simulink model "AUAV_V3_TestSensors"  (R2015a)
settings: Solver=FixedStepDiscrete  StartTime=0.0  StopTime=10.0  FixedStep=T  RelTol=1e-3
PreLoadFcn:
  | %T = 0.0025;
  | MavlinkBus;
  | mcuInit;
  | % Baro Altitude Computation
  | % =========================
  | basePressure = 98192.64;
  | baseTemp = 288.215;
  | lapseRate = -0.00198122;
  | baseHeight = 0;
undefined symbols (not defined in the file): A0, A14, A15, A2, A3, A4, A5, A6, accBiasRateLimit, apSampleTime, B0, bankCommandLimit, barAdjust, baroCutoff, baroCutTemp, baroOffset, baroScale, barTGain1, barTGain2, barTMean1, barTMean2, bda, bde, bdr, bdt, bICda, bICde, bICdr, bICdt, cubeAccelGain16405, cubeGyroGain16405, cubeMagGain16405, D0, D11, D7, D8, daLimit, data, daTrimMax, daTrimMin, deLimit, derivativesConstant, deTrimMax, deTrimMin, drLimit, drTrimMax, drTrimMin, dtLimit, dtTrimMax, dtTrimMin, F2, F3, G0, G13, G15, gaind, GS_location, gyroBiasRateLimit, IC1max, imuOffset_xacc ... (+77)
libraries: MCHP_Blockset x158, simulink x84, SLUGS_Library x31, aerolibconvert2 x6, aerolibutil x4, aerolibtransform2 x3, dspmtrx3 x2, aerolibobsolete x2
(part 17 of 23)

== system AUAV_V3_TestSensors/Sensor_Data_Adapter/Sensor Suite/Low Pass Filtering,Temperature Compensation and Calibration ==
  Baro raw : Inport
  Pitot raw : Inport  Port=2
  Power Raw : Inport  Port=3
  Therm Raw : Inport  Port=4
  Baro Altimeter : Subsystem
  Barometer Unit Conversion : Subsystem  mask{bias=baroOffset, gains=baroScale}
      mask prompts: bias "Initial Bias"; gains "Initial Gains"
      mask help: Convert Analog readings to units
  Data Type Conversion1 : DataTypeConversion  OutDataTypeStr=single
  Data Type Conversion{3,5..6,19} (4 alike) : DataTypeConversion  OutDataTypeStr=double
  Data Type Conversion4 : DataTypeConversion  OutDataTypeStr=single
  Data Type Conversion8 : DataTypeConversion  OutDataTypeStr=uint16
  Pitot Unit Conversion : Subsystem  mask{bias=pitotOffset, gains=pitotScale}
      mask prompts: bias "Initial Bias"; gains "Initial Gains"
      mask help: Convert Analog readings to units
  Power Unit Conversion : Subsystem  mask{bias=powerOffset, gains=powerScale}
      mask prompts: bias "Initial Bias"; gains "Initial Gains"
      mask help: Convert Analog readings to units
  Temp Compensate Accel X1 : Subsystem
  Temp Compensate Baro : Subsystem
  Thermistor Unit Conversion : Subsystem  mask{bias=tempOffset, gains=tempScale}
      mask prompts: bias "Initial Bias"; gains "Initial Gains"
      mask help: Convert Analog readings to units
  "Tustin Lowpass, Auto Initial Condition1" : Subsystem  mask(Tustin1stOrderLowpassAutoInitialCondition){f=lowRateSensorCutoff, T=apSampleTime}
      mask prompts: f "Lowpass Frequency"; T "Sample Time"
      mask help: Takes a 3db rolloff frequency (in Hz, NOT radians/s) and a sample time. Performs a symbolic Tustin conversion and implements in a discrete filter. The initial output of the filter is set by the first sample.
      mask Help: Enter the desired 3db rolloff frequency in Hz and the sample time. Initial conditions are sampled automatically.
      mask Display: fprintf('%.2f Hz lowpass',f)
  "Tustin Lowpass, Auto Initial Condition2" : Subsystem  mask(Tustin1stOrderLowpassAutoInitialCondition){f=lowRateSensorCutoff, T=apSampleTime}
      mask prompts: f "Lowpass Frequency"; T "Sample Time"
      mask help: Takes a 3db rolloff frequency (in Hz, NOT radians/s) and a sample time. Performs a symbolic Tustin conversion and implements in a discrete filter. The initial output of the filter is set by the first sample.
      mask Help: Enter the desired 3db rolloff frequency in Hz and the sample time. Initial conditions are sampled automatically.
      mask Display: fprintf('%.2f Hz lowpass',f)
  "Tustin Lowpass, Auto Initial Condition3" : Subsystem  mask(Tustin1stOrderLowpassAutoInitialCondition){f=pressureSensorCutoff, T=apSampleTime}
      mask prompts: f "Lowpass Frequency"; T "Sample Time"
      mask help: Takes a 3db rolloff frequency (in Hz, NOT radians/s) and a sample time. Performs a symbolic Tustin conversion and implements in a discrete filter. The initial output of the filter is set by the first sample.
      mask Help: Enter the desired 3db rolloff frequency in Hz and the sample time. Initial conditions are sampled automatically.
      mask Display: fprintf('%.2f Hz lowpass',f)
  "Tustin Lowpass, Auto Initial Condition4" : Subsystem  mask(Tustin1stOrderLowpassAutoInitialCondition){f=pressureSensorCutoff, T=apSampleTime}
      mask prompts: f "Lowpass Frequency"; T "Sample Time"
      mask help: Takes a 3db rolloff frequency (in Hz, NOT radians/s) and a sample time. Performs a symbolic Tustin conversion and implements in a discrete filter. The initial output of the filter is set by the first sample.
      mask Help: Enter the desired 3db rolloff frequency in Hz and the sample time. Initial conditions are sampled automatically.
      mask Display: fprintf('%.2f Hz lowpass',f)
  "[0.001  maxDynPress]" : Saturate  UpperLimit=maxDynPressure  LowerLimit=0.001
  Baro Alt (m) : Outport
  Pitot (Pa) : Outport  Port=2
  Static (Pa) : Outport  Port=3
  Temp (0.1 C) : Outport  Port=4
  Power (V) : Outport  Port=5
  wires:
  "Tustin Lowpass, Auto Initial Condition1"/1(Out1) -> Thermistor Unit Conversion/1(Raw)
  "[0.001  maxDynPress]"/1 -> Pitot (Pa)/1
  Data Type Conversion19/1 -> "Tustin Lowpass, Auto Initial Condition4"/1(In1)
  Data Type Conversion3/1 -> "Tustin Lowpass, Auto Initial Condition3"/1(In1)
  "Tustin Lowpass, Auto Initial Condition3"/1(Out1) -> Data Type Conversion4/1
  Data Type Conversion5/1 -> "Tustin Lowpass, Auto Initial Condition1"/1(In1)
  Therm Raw/1 -> Data Type Conversion5/1
  Barometer Unit Conversion/1(Comp) -> Static (Pa)/1, Baro Altimeter/1(Static (Pa))
  Data Type Conversion4/1 -> Pitot Unit Conversion/1(Raw)
  "Tustin Lowpass, Auto Initial Condition4"/1(Out1) -> Data Type Conversion1/1
  Data Type Conversion1/1 -> Barometer Unit Conversion/1(Raw)
  Thermistor Unit Conversion/1(Comp) -> Temp (0.1 C)/1, [Temp]
  Data Type Conversion6/1 -> "Tustin Lowpass, Auto Initial Condition2"/1(In1)
  Power Raw/1 -> Data Type Conversion6/1
  "Tustin Lowpass, Auto Initial Condition2"/1(Out1) -> Power Unit Conversion/1(Raw)
  Data Type Conversion8/1 -> Power (V)/1
  Baro Altimeter/1(Altitude) -> Baro Alt (m)/1
  Pitot Unit Conversion/1(Comp) -> "[0.001  maxDynPress]"/1
  Power Unit Conversion/1(Comp) -> Data Type Conversion8/1
  Temp Compensate Baro/1(Baro_c) -> Data Type Conversion19/1
  [Temp] -> Temp Compensate Baro/1(Temp)
  Baro raw/1 -> Temp Compensate Baro/2(Baro)
  [Temp] -> Temp Compensate Accel X1/1(Temp)
  Pitot raw/1 -> Temp Compensate Accel X1/2(Dynamic)
  Temp Compensate Accel X1/1(Baro_c) -> Data Type Conversion3/1

== system AUAV_V3_TestSensors/Trim Vals [updated 4.28.16]/Control Surface Input/2 sec  tau ==
  In1 : Inport
  Constant : Constant  Value=T
  Constant1 : Constant  Value=f
  Embedded MATLAB Function : MATLAB Function  TreatAsAtomicUnit=on
  Out1 : Outport
  wires:
  In1/1 -> Embedded MATLAB Function/1(u)
  Embedded MATLAB Function/1(y) -> Out1/1
  Constant1/1 -> Embedded MATLAB Function/3(f)
  Constant/1 -> Embedded MATLAB Function/2(T)

== system AUAV_V3_TestSensors/Trim Vals [updated 4.28.16]/Control Surface Input/2 sec  tau1 ==
  In1 : Inport
  Constant : Constant  Value=T
  Constant1 : Constant  Value=f
  Embedded MATLAB Function : MATLAB Function  TreatAsAtomicUnit=on
  Out1 : Outport
  wires:
  Constant/1 -> Embedded MATLAB Function/2(T)
  Constant1/1 -> Embedded MATLAB Function/3(f)
  Embedded MATLAB Function/1(y) -> Out1/1
  In1/1 -> Embedded MATLAB Function/1(u)

== system AUAV_V3_TestSensors/Trim Vals [updated 4.28.16]/Detect Transition High to Low/Subsystem ==
  WP Fly : Inport
  C Function Call : MCHP_Blockset/User Functions/C Function Call  ParseFilesChkbx=off  ListFunctions1=Custom Function  Function1=extern uint8_T justEnabled(uint8_T u1, uint8_T u2);  AddHeaderDeclaration=on  Function1Type=when block is updated (default)  Fct1BlockIn=u1, u2  FctReturnBlockOut=on  DataCollected=0  ORDERING=None  SampleTime=-1  MCHP_MASTERLINK=|  PinDigitalInput=[]  PinDigitalOutput=[]  PinAnalogInput=[]
      | AUAV_V3_TestSensors/Microchip Master
      | AUAV V3 Board
      | Busy Flag on D2 (RA6)
  Data Type Conversion1 : DataTypeConversion  OutDataTypeStr=uint8  SampleTime=apSampleTime
  Index : Constant  Value=2  OutDataTypeStr=uint8
  Just Enab : Outport
  wires:
  WP Fly/1 -> Data Type Conversion1/1
  Data Type Conversion1/1 -> C Function Call/1
  Index/1 -> C Function Call/2
  C Function Call/1 -> Just Enab/1

== system AUAV_V3_TestSensors/Trim Vals [updated 4.28.16]/Grab I.C./Convert to Microseconds  ==
  IC : Inport
  Convert to Microseconds : Gain  Gain=0.2
  Data Type Conversion : DataTypeConversion  OutDataTypeStr=uint16
  uS : Outport
  wires:
  Convert to Microseconds/1 -> Data Type Conversion/1
  IC/1 -> Convert to Microseconds/1
  Data Type Conversion/1 -> uS/1

== system AUAV_V3_TestSensors/Trim Vals [updated 4.28.16]/Grab I.C./Convert to Microseconds 1 ==
  IC : Inport
  Convert to Microseconds : Gain  Gain=0.2
  Data Type Conversion : DataTypeConversion  OutDataTypeStr=uint16
  uS : Outport
  wires:
  Data Type Conversion/1 -> uS/1
  IC/1 -> Convert to Microseconds/1
  Convert to Microseconds/1 -> Data Type Conversion/1

== system AUAV_V3_TestSensors/Trim Vals [updated 4.28.16]/Grab I.C./Convert to Microseconds 2 ==
  IC : Inport
  Convert to Microseconds : Gain  Gain=0.2
  Data Type Conversion : DataTypeConversion  OutDataTypeStr=uint16
  uS : Outport
  wires:
  Convert to Microseconds/1 -> Data Type Conversion/1
  IC/1 -> Convert to Microseconds/1
  Data Type Conversion/1 -> uS/1

== system AUAV_V3_TestSensors/Trim Vals [updated 4.28.16]/Grab I.C./Convert to Microseconds 3 ==
  IC : Inport
  Convert to Microseconds : Gain  Gain=0.2
  Data Type Conversion : DataTypeConversion  OutDataTypeStr=uint16
  uS : Outport
  wires:
  Data Type Conversion/1 -> uS/1
  IC/1 -> Convert to Microseconds/1
  Convert to Microseconds/1 -> Data Type Conversion/1

== system AUAV_V3_TestSensors/Trim Vals [updated 4.28.16]/Grab I.C./Convert to Rad ==
  IC : Inport
  Add : Sum
  Constant1 : Constant  Value=slopem
  Constant2 : Constant  Value=interceptb
  Data Type Conversion : DataTypeConversion  OutDataTypeStr=single
  Divide : Product
  Angle (rad) : Outport
  wires:
  Data Type Conversion/1 -> Angle (rad)/1
  IC/1 -> Divide/1
  Constant2/1 -> Add/2
  Divide/1 -> Add/1
  Add/1 -> Data Type Conversion/1
  Constant1/1 -> Divide/2

== system AUAV_V3_TestSensors/Trim Vals [updated 4.28.16]/Grab I.C./Convert to Rad1 ==
  IC : Inport
  Add : Sum
  Constant1 : Constant  Value=slopem
  Constant2 : Constant  Value=interceptb
  Data Type Conversion : DataTypeConversion  OutDataTypeStr=single
  Divide : Product
  Angle (rad) : Outport
  wires:
  Constant1/1 -> Divide/2
  Add/1 -> Data Type Conversion/1
  Divide/1 -> Add/1
  Constant2/1 -> Add/2
  IC/1 -> Divide/1
  Data Type Conversion/1 -> Angle (rad)/1

== system AUAV_V3_TestSensors/Trim Vals [updated 4.28.16]/Grab I.C./Convert to Rad2 ==
  IC : Inport
  Add : Sum
  Constant1 : Constant  Value=slopem
  Constant2 : Constant  Value=interceptb
  Data Type Conversion : DataTypeConversion  OutDataTypeStr=single
  Divide : Product
  Angle (rad) : Outport
  wires:
  Data Type Conversion/1 -> Angle (rad)/1
  IC/1 -> Divide/1
  Constant2/1 -> Add/2
  Divide/1 -> Add/1
  Add/1 -> Data Type Conversion/1
  Constant1/1 -> Divide/2

== system AUAV_V3_TestSensors/Trim Vals [updated 4.28.16]/Grab I.C./Convert to Rad3 ==
  IC : Inport
  Add : Sum
  Constant1 : Constant  Value=slopem
  Constant2 : Constant  Value=interceptb
  Data Type Conversion : DataTypeConversion  OutDataTypeStr=single
  Divide : Product
  Angle (rad) : Outport
  wires:
  Constant1/1 -> Divide/2
  Add/1 -> Data Type Conversion/1
  Divide/1 -> Add/1
  Constant2/1 -> Add/2
  IC/1 -> Divide/1
  Data Type Conversion/1 -> Angle (rad)/1

== system AUAV_V3_TestSensors/Update PWM Commands and Send Telemetry [updated 4.27.16]/Generate PWM Signals Based on the Control Type/If  Control Type Is Manual ==
  Pilot (IC) : Inport
  Action Port : ActionPort  ActionType=then
  Gain4 : Gain  Gain=0.5  OutDataTypeStr=Inherit: Same as input
  PWM : Outport
  wires:
  Pilot (IC)/1 -> Gain4/1
  Gain4/1 -> PWM/1

== system AUAV_V3_TestSensors/Update PWM Commands and Send Telemetry [updated 4.27.16]/Generate PWM Signals Based on the Control Type/If  Control Type Is Passthrough ==
  Pilot (IC) : Inport
  Action Port : ActionPort  ActionType=elseif
  Gain4 : Gain  Gain=0.5  OutDataTypeStr=Inherit: Same as input
  PWM (abs) : Outport
  wires:
  Gain4/1 -> PWM (abs)/1
  Pilot (IC)/1 -> Gain4/1

== system AUAV_V3_TestSensors/Update PWM Commands and Send Telemetry [updated 4.27.16]/Generate PWM Signals Based on the Control Type/If  Control Type Is Selective Passthrough ==
  PWM(rad) : Inport
  Pilot (IC) : Inport  Port=2
  Action Port : ActionPort  ActionType=elseif
  Convert to PWM : Subsystem  mask{slopem=mde / 2., interceptb=bde / 2.}
      mask prompts: slopem "Slope"; interceptb "Intercept"
  Convert to PWM1 : Subsystem  mask{slopem=mdt / 2., interceptb=bdt / 2.}
      mask prompts: slopem "Slope"; interceptb "Intercept"
  Convert to PWM2 : Subsystem  mask{slopem=mda / 2., interceptb=bda / 2.}
      mask prompts: slopem "Slope"; interceptb "Intercept"
  Convert to PWM3 : Subsystem  mask{slopem=mdr / 2., interceptb=bdr / 2.}
      mask prompts: slopem "Slope"; interceptb "Intercept"
  Demux : Demux
  Demux1 : Demux
  Demux2 : Demux
  Gain{,1..3} (4 alike) : Gain  Gain=0.5  OutDataTypeStr=Inherit: Same as input
  Initialize Control MCU : MCHP_Blockset/User Functions/C Function Call  ParseFilesChkbx=off  ListFunctions1=Custom Function  Function1=extern void getPassValues(uint8_T* pasVals)  AddHeaderDeclaration=on  Function1Type=when block is updated (default)  FctReturnBlockOut=on  Fct1BlockOut=pasVals  DataCollected=0  ORDERING=None  SampleTime=.01  MCHP_MASTERLINK=|  PinDigitalInput=[]  PinDigitalOutput=[]  PinAnalogInput=[]
      | AUAV_V3_TestSensors/Microchip Master
      | AUAV V3 Board
      | Busy Flag on D2 (RA6)
  Switch{,1..3} (4 alike) : Switch  Threshold=0.5
  myMux Fun1 : MATLAB Function  TreatAsAtomicUnit=on
  PWM : Outport
  wires:
  Switch/1 -> myMux Fun1/1(u1)
  Switch1/1 -> myMux Fun1/2(u2)
  Switch2/1 -> myMux Fun1/3(u3)
  Switch3/1 -> myMux Fun1/4(u4)
  Initialize Control MCU/1 -> Demux/1
  Demux/4 -> Switch/2
  Demux/3 -> Switch1/2
  Demux/2 -> Switch2/2
  Demux/1 -> Switch3/2
  Demux1/1 -> Convert to PWM1/1(" Angle(rad)")
  Demux1/2 -> Convert to PWM2/1(" Angle(rad)")
  Demux1/3 -> Convert to PWM3/1(" Angle(rad)")
  Demux1/4 -> Convert to PWM/1(" Angle(rad)")
  PWM(rad)/1 -> Demux1/1
  Convert to PWM1/1(PWM) -> Switch/3
  Convert to PWM2/1(PWM) -> Switch1/3
  Convert to PWM3/1(PWM) -> Switch2/3
  Convert to PWM/1(PWM) -> Switch3/3
  Demux2/1 -> Gain/1
  Demux2/2 -> Gain1/1
  Demux2/3 -> Gain2/1
  Demux2/4 -> Gain3/1
  Pilot (IC)/1 -> Demux2/1
  Gain/1 -> Switch/1
  Gain1/1 -> Switch1/1
  Gain2/1 -> Switch2/1
  Gain3/1 -> Switch3/1
  myMux Fun1/1(y) -> PWM/1

== system AUAV_V3_TestSensors/Update PWM Commands and Send Telemetry [updated 4.27.16]/Generate PWM Signals Based on the Control Type/If  Control Type Is Wp, ISR, LP or  Mid Lvl Cmds ==
  PWM(rad) : Inport
  Action Port : ActionPort  ActionType=elseif
  Convert to PWM : Subsystem  mask{slopem=mde / 2., interceptb=bde / 2.}
      mask prompts: slopem "Slope"; interceptb "Intercept"
  Convert to PWM1 : Subsystem  mask{slopem=mdt / 2., interceptb=bdt / 2.}
      mask prompts: slopem "Slope"; interceptb "Intercept"
  Convert to PWM2 : Subsystem  mask{slopem=mda / 2., interceptb=bda / 2.}
      mask prompts: slopem "Slope"; interceptb "Intercept"
  Convert to PWM3 : Subsystem  mask{slopem=mdr / 2., interceptb=bdr / 2.}
      mask prompts: slopem "Slope"; interceptb "Intercept"
  Demux : Demux
  myMux Fun1 : MATLAB Function  TreatAsAtomicUnit=on
  PWM (abs) : Outport
  wires:
  Convert to PWM1/1(PWM) -> myMux Fun1/1(u1)
  Convert to PWM2/1(PWM) -> myMux Fun1/2(u2)
  Convert to PWM3/1(PWM) -> myMux Fun1/3(u3)
  Convert to PWM/1(PWM) -> myMux Fun1/4(u4)
  Demux/1 -> Convert to PWM1/1(" Angle(rad)")
  Demux/2 -> Convert to PWM2/1(" Angle(rad)")
  Demux/3 -> Convert to PWM3/1(" Angle(rad)")
  Demux/4 -> Convert to PWM/1(" Angle(rad)")
  PWM(rad)/1 -> Demux/1
  myMux Fun1/1(y) -> PWM (abs)/1

== system AUAV_V3_TestSensors/Barometer_Driver/Baro Altimeter/Initial Baro Bias/Low Pass8 ==
  In1 : Inport
  Discrete Zero-Pole : DiscreteZeroPole  Zeros=zerosd  Poles=polesd  Gain=gaind  SampleTime=SampleTime
  Out1 : Outport
  wires:
  Discrete Zero-Pole/1 -> Out1/1
  In1/1 -> Discrete Zero-Pole/1

== system AUAV_V3_TestSensors/Inner Loop// Navigation/L1 Output Feedback Controller With Projection Operator/Control Law/Compute Coef ==
  a : Inport
  Enable : EnablePort
  -T : Gain  Gain=-apSampleTime  SampleTime=apSampleTime
  1-c : Sum  Inputs=-+  OutDataTypeStr=single  SampleTime=apSampleTime
  Constant : Constant
  dsPIC_exp : Subsystem  AncestorBlock=SLUGS_Library/dsPIC_exp
  b : Outport
  c : Outport  Port=2
  wires:
  -T/1 -> dsPIC_exp/1(u)
  dsPIC_exp/1(exp(u)) -> 1-c/1, c/1  "c"
  Constant/1 -> 1-c/2
  1-c/1 -> b/1
  a/1 -> -T/1

== system AUAV_V3_TestSensors/Inner Loop// Navigation/L1 Output Feedback Controller With Projection Operator/Control Law/Detect Change ==
  Data : Inport
  Abs1 : Abs  SampleTime=apSampleTime
  Difference1 : simulink/Discrete/Difference  ICPrevInput=0.0  InputProcessing=Inherited  OutMin=[]  OutMax=[]  OutDataType=sfix(16)  OutScaling=2^-10  DoSatur=off
  Saturation1 : Saturate  UpperLimit=1  LowerLimit=0  SampleTime=apSampleTime
  change? : Outport
  wires:
  Difference1/1 -> Abs1/1
  Abs1/1 -> Saturation1/1
  Data/1 -> Difference1/1
  Saturation1/1 -> change?/1

== system AUAV_V3_TestSensors/Inner Loop// Navigation/L1 Output Feedback Controller With Projection Operator/Projection Operator/Enabled Subsystem ==
  In1 : Inport
  Enable : EnablePort
  Out1 : Outport
  wires:
  In1/1 -> Out1/1

== system AUAV_V3_TestSensors/Inner Loop// Navigation/L1 Output Feedback Controller With Projection Operator/Projection Operator/Enabled Subsystem1 ==
  y : Inport
  f_the : Inport  Port=2
  grad : Inport  Port=3
  Enable : EnablePort
  Constant : Constant  OutDataTypeStr=single
  Divide1 : Product  OutDataTypeStr=single
  Divide2 : Product  OutDataTypeStr=single
  Sign : Signum
  Subtract : Sum  Inputs=+-  OutDataTypeStr=single
  Out1 : Outport
  wires:
  Divide1/1 -> Subtract/2
  grad/1 -> Sign/1
  Sign/1 -> Divide1/2
  Constant/1 -> Subtract/1
  f_the/1 -> Divide1/1
  Subtract/1 -> Divide2/2
  y/1 -> Divide2/1
  Divide2/1 -> Out1/1

== system AUAV_V3_TestSensors/Inner Loop// Navigation/L1 Output Feedback Controller With Projection Operator/Projection Operator/F(theta) ==
  Theta Max : Inport
  Eps 0 : Inport  Port=2
  Theta : Inport  Port=3
  Constant : Constant  Value=2  OutDataTypeStr=single
  Divide : Product  OutDataTypeStr=single
  Divide1 : Product  OutDataTypeStr=single
  Divide2 : Product  OutDataTypeStr=single
  Divide3 : Product  Inputs=*/  OutDataTypeStr=single
  Divide4 : Product  Inputs=/**  OutDataTypeStr=single
  Subtract : Sum  Inputs=+-  OutDataTypeStr=single
  "Theta " : InportShadow  Port=3
  f_theta : Outport
  dif_f_theta : Outport  Port=2
  wires:
  Theta/1 -> Divide/1, Divide/2
  Theta Max/1 -> Divide1/2, Divide1/1
  Divide/1 -> Subtract/1
  Divide1/1 -> Subtract/2, Divide2/1
  Eps 0/1 -> Divide2/2
  Subtract/1 -> Divide3/1
  Divide2/1 -> Divide3/2, Divide4/1
  Divide3/1 -> f_theta/1
  Constant/1 -> Divide4/3
  "Theta "/1 -> Divide4/2
  Divide4/1 -> dif_f_theta/1

== system AUAV_V3_TestSensors/Inner Loop// Navigation/L1 Output Feedback Controller With Projection Operator/State Predictor/Compute Coef ==
  a : Inport
  Enable : EnablePort
  -T : Gain  Gain=-apSampleTime  SampleTime=apSampleTime
  1-c : Sum  Inputs=-+  OutDataTypeStr=single
  Constant : Constant
  dsPIC_exp : Subsystem  AncestorBlock=SLUGS_Library/dsPIC_exp
  b : Outport
  c : Outport  Port=2
  wires:
  a/1 -> -T/1
  1-c/1 -> b/1
  Constant/1 -> 1-c/2
  dsPIC_exp/1(exp(u)) -> c/1, 1-c/1  "c"
  -T/1 -> dsPIC_exp/1(u)

== system AUAV_V3_TestSensors/Inner Loop// Navigation/L1 Output Feedback Controller With Projection Operator/State Predictor/Detect Change ==
  Data : Inport
  Abs1 : Abs  SampleTime=apSampleTime
  Difference1 : simulink/Discrete/Difference  ICPrevInput=0.0  InputProcessing=Inherited  OutMin=[]  OutMax=[]  OutDataType=sfix(16)  OutScaling=2^-10  DoSatur=off
  Saturation1 : Saturate  UpperLimit=1  LowerLimit=0  SampleTime=apSampleTime
  change? : Outport
  wires:
  Saturation1/1 -> change?/1
  Data/1 -> Difference1/1
  Abs1/1 -> Saturation1/1
  Difference1/1 -> Abs1/1

== system AUAV_V3_TestSensors/Inner Loop// Navigation/L1 Output Feedback Controller With Projection Operator/Trapezoidal Integrator/Protect NaNs ==
  In1 : Inport
  Integer Delay3 : Delay  DelayLength=1  InputProcessing=Inherited  SampleTime=T
  Relational Operator2 : RelationalOperator  Operator===  OutDataTypeStr=uint(8)
  Switch3 : Switch  Criteria=u2 > Threshold  Threshold=0.3  SampleTime=.01
  Out1 : Outport
  wires:
  Relational Operator2/1 -> Switch3/2
  In1/1 -> Switch3/1, Relational Operator2/1, Relational Operator2/2
  Switch3/1 -> Integer Delay3/1, Out1/1
  Integer Delay3/1 -> Switch3/3

== system AUAV_V3_TestSensors/Inner Loop// Navigation/L1 Output Feedback Controller With Projection Operator/Trapezoidal Integrator/Protect NaNs1 ==
  In1 : Inport
  Integer Delay3 : Delay  DelayLength=1  InputProcessing=Inherited  SampleTime=T
  Relational Operator2 : RelationalOperator  Operator===  OutDataTypeStr=uint(8)
  Switch3 : Switch  Criteria=u2 > Threshold  Threshold=0.3  SampleTime=.01
  Out1 : Outport
  wires:
  Integer Delay3/1 -> Switch3/3
  Switch3/1 -> Out1/1, Integer Delay3/1
  In1/1 -> Relational Operator2/2, Relational Operator2/1, Switch3/1
  Relational Operator2/1 -> Switch3/2

== system AUAV_V3_TestSensors/Inner Loop// Navigation/Lateral Channel Encaps [updated 4.28.16]/Lateral Channel/0.016 sec  tau ==
  In1 : Inport
  Constant : Constant  Value=T
  Constant1 : Constant  Value=f
  Embedded MATLAB Function : MATLAB Function  TreatAsAtomicUnit=on
  Out1 : Outport
  wires:
  In1/1 -> Embedded MATLAB Function/1(u)
  Embedded MATLAB Function/1(y) -> Out1/1
  Constant1/1 -> Embedded MATLAB Function/3(f)
  Constant/1 -> Embedded MATLAB Function/2(T)

== system AUAV_V3_TestSensors/Inner Loop// Navigation/Lateral Channel Encaps [updated 4.28.16]/Lateral Channel/Protect NaNs ==
  In1 : Inport
  Integer Delay3 : Delay  DelayLength=1  InputProcessing=Inherited
  Relational Operator2 : RelationalOperator  Operator===  OutDataTypeStr=uint(8)
  Switch3 : Switch  Criteria=u2 > Threshold  Threshold=0.3
  Out1 : Outport
  wires:
  Integer Delay3/1 -> Switch3/3
  Switch3/1 -> Out1/1, Integer Delay3/1
  In1/1 -> Relational Operator2/2, Relational Operator2/1, Switch3/1
  Relational Operator2/1 -> Switch3/2

== system AUAV_V3_TestSensors/Inner Loop// Navigation/Lateral Channel Encaps [updated 4.28.16]/Lateral Channel/Protect NaNs2 ==
  In1 : Inport
  Integer Delay3 : Delay  DelayLength=1  InputProcessing=Inherited  SampleTime=T
  Relational Operator2 : RelationalOperator  Operator===  OutDataTypeStr=uint(8)
  Switch3 : Switch  Criteria=u2 > Threshold  Threshold=0.3  SampleTime=.01
  Out1 : Outport
  wires:
  Integer Delay3/1 -> Switch3/3
  Switch3/1 -> Out1/1, Integer Delay3/1
  In1/1 -> Relational Operator2/2, Relational Operator2/1, Switch3/1
  Relational Operator2/1 -> Switch3/2

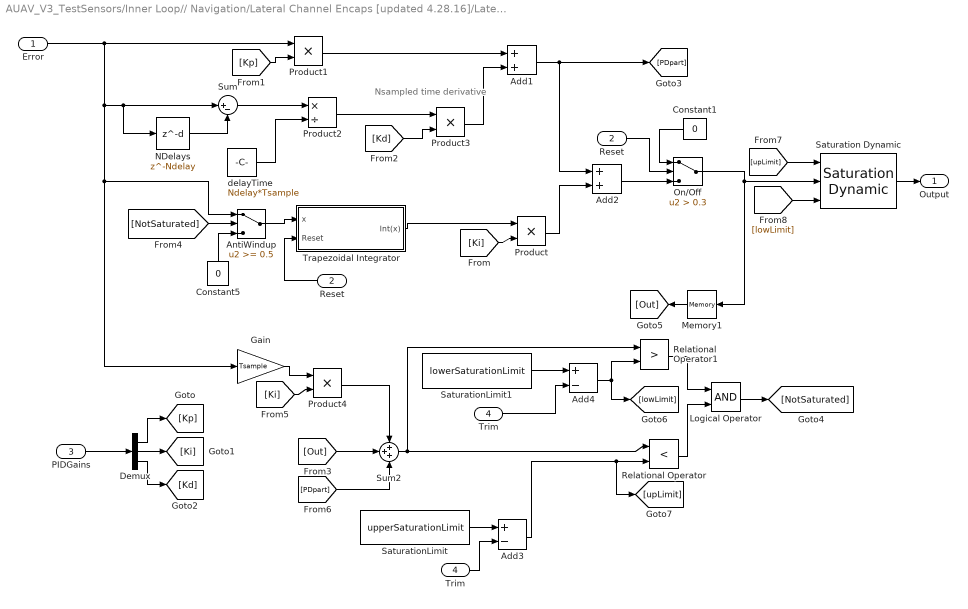
== system AUAV_V3_TestSensors/Inner Loop// Navigation/Lateral Channel Encaps [updated 4.28.16]/Lateral Channel/Roll Control [PID] ==
  note: Nsampled time derivative
  Error : Inport
  Reset : Inport  Port=2
  PIDGains : Inport  Port=3
  Trim : Inport  Port=4
  Add1 : Sum
  Add2 : Sum  OutDataTypeStr=single
  Add3 : Sum  Inputs=+-  OutDataTypeStr=single
  Add4 : Sum  Inputs=+-  OutDataTypeStr=single
  AntiWindup : Switch  Threshold=0.5
  Constant1 : Constant  Value=0  OutDataTypeStr=single
  Constant5 : Constant  Value=0  OutDataTypeStr=single
  Demux : Demux  Outputs=3
  Gain : Gain  Gain=Tsample
  Logical Operator : Logic  AllPortsSameDT=off  OutDataTypeStr=boolean
  Memory1 : Memory  InheritSampleTime=on
  NDelays : Delay  DelayLength=Ndelay  InputProcessing=Inherited  SampleTime=Tsample
  On/Off : Switch  Criteria=u2 > Threshold  Threshold=0.3
  Product{,1,3..4} (4 alike) : Product  RndMeth=Zero
  Product2 : Product  Inputs=*/  RndMeth=Zero
  Relational Operator : RelationalOperator  Operator=<  OutDataTypeStr=boolean
  Relational Operator1 : RelationalOperator  Operator=>  OutDataTypeStr=boolean
  "Reset " : InportShadow  Port=2
  Saturation Dynamic : simulink/Discontinuities/Saturation Dynamic  OutMin=[]  OutMax=[]  OutDataTypeStr=Inherit: Same as second input  OutDataType=fixdt(1, 16)  OutScaling=2^-10  DoSatur=off
  SaturationLimit : Constant  Value=upperSaturationLimit  OutDataTypeStr=single
  SaturationLimit1 : Constant  Value=lowerSaturationLimit  OutDataTypeStr=single
  Sum : Sum  Inputs=|+-
  Sum2 : Sum  Inputs=+++
  Trapezoidal Integrator : Subsystem  mask{T=Tsample}
      mask prompts: T "Sample Time"
  "Trim " : InportShadow  Port=4
  delayTime : Constant  Value=Ndelay*Tsample  OutDataTypeStr=single
  Output : Outport
  wires:
  On/Off/1 -> Memory1/1, Saturation Dynamic/2
  Constant1/1 -> On/Off/1
  "Reset "/1 -> On/Off/2
  Add2/1 -> On/Off/3
  [NotSaturated] -> AntiWindup/2
  Saturation Dynamic/1 -> Output/1
  Product2/1 -> Product3/1
  [Kd] -> Product3/2
  delayTime/1 -> Product2/2
  Sum/1 -> Product2/1
  NDelays/1 -> Sum/2
  [Kp] -> Product1/2
  Trapezoidal Integrator/1(Int(x)) -> Product/1
  [Ki] -> Product/2
  Error/1 -> Product1/1, Sum/1, NDelays/1, AntiWindup/1, Gain/1
  AntiWindup/1 -> Trapezoidal Integrator/1(x)
  Constant5/1 -> AntiWindup/3
  Demux/3 -> [Kd]
  Demux/2 -> [Ki]
  Demux/1 -> [Kp]
  PIDGains/1 -> Demux/1
  Memory1/1 -> [Out]
  Reset/1 -> Trapezoidal Integrator/2(Reset)
  Product1/1 -> Add1/1
  Product3/1 -> Add1/2
  Add1/1 -> [PDpart], Add2/1
  Product/1 -> Add2/2
  [PDpart] -> Sum2/3
  Product4/1 -> Sum2/1
  Gain/1 -> Product4/1
  [Ki] -> Product4/2
  Sum2/1 -> Relational Operator/1, Relational Operator1/1
  [Out] -> Sum2/2
  Add3/1 -> Relational Operator/2, [upLimit]
  Relational Operator/1 -> Logical Operator/2
  Relational Operator1/1 -> Logical Operator/1
  Logical Operator/1 -> [NotSaturated]
  Trim/1 -> Add3/2
  SaturationLimit/1 -> Add3/1
  Add4/1 -> Relational Operator1/2, [lowLimit]
  SaturationLimit1/1 -> Add4/1
  "Trim "/1 -> Add4/2
  [upLimit] -> Saturation Dynamic/1
  [lowLimit] -> Saturation Dynamic/3

== system AUAV_V3_TestSensors/Inner Loop// Navigation/Lateral Channel Encaps [updated 4.28.16]/Lateral Channel/Sideslip Compensation ==
  phi_m : Inport
  r_m : Inport  Port=2
  U_m : Inport  Port=3
  Enable : EnablePort  StatesWhenEnabling=reset
  Bank to Psi Dot : Subsystem  AncestorBlock=SLUGS_Library/Navigation/Bank to Psi Dot
  Constant : Constant  Value=0.3  OutDataTypeStr=single
  Low Pass : Subsystem
      mask Display:
      | droots([],'-a','a')
      | port_label('input',1,'a')
      | port_label('input',2,'u')
      | port_label('output',1,'y')
  Protect NaNs2 : Subsystem
  Subtract : Sum  Inputs=+-
  psi_dot to Bank : Subsystem  AncestorBlock=SLUGS_Library/Navigation/psi_dot to Bank
  bankComp : Outport  OutputWhenDisabled=reset  InitialOutput=0
  wires:
  Protect NaNs2/1(Out1) -> Low Pass/2(u)
  phi_m/1 -> Bank to Psi Dot/1(phi_c)
  r_m/1 -> Subtract/2
  U_m/1 -> Bank to Psi Dot/2(U_m), psi_dot to Bank/2(U_m)
  Bank to Psi Dot/1(psi_dot_c) -> Subtract/1  "coord turn"
  Subtract/1 -> psi_dot to Bank/1(psi_dot_c)  "turn rate error"
  psi_dot to Bank/1(phi_c) -> Protect NaNs2/1(In1)  "phi error"
  Low Pass/1(y) -> bankComp/1
  Constant/1 -> Low Pass/1(a)

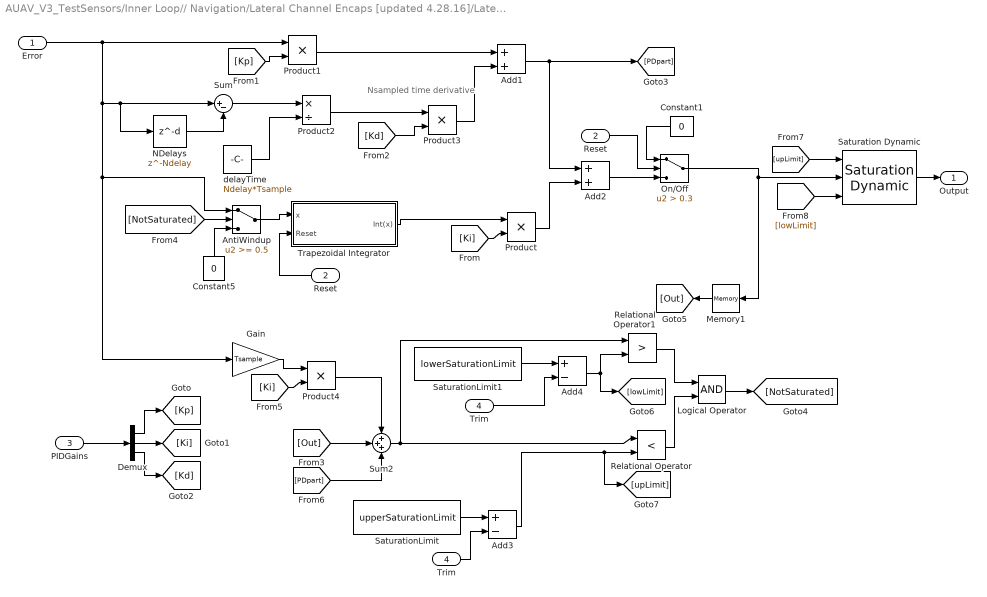
== system AUAV_V3_TestSensors/Inner Loop// Navigation/Lateral Channel Encaps [updated 4.28.16]/Lateral Channel/Yaw Damper [PID] ==
  note: Nsampled time derivative
  Error : Inport
  Reset : Inport  Port=2
  PIDGains : Inport  Port=3
  Trim : Inport  Port=4
  Add1 : Sum
  Add2 : Sum  OutDataTypeStr=single
  Add3 : Sum  Inputs=+-  OutDataTypeStr=single
  Add4 : Sum  Inputs=+-  OutDataTypeStr=single
  AntiWindup : Switch  Threshold=0.5
  Constant1 : Constant  Value=0  OutDataTypeStr=single
  Constant5 : Constant  Value=0  OutDataTypeStr=single
  Demux : Demux  Outputs=3
  Gain : Gain  Gain=Tsample
  Logical Operator : Logic  AllPortsSameDT=off  OutDataTypeStr=boolean
  Memory1 : Memory  InheritSampleTime=on
  NDelays : Delay  DelayLength=Ndelay  InputProcessing=Inherited  SampleTime=Tsample
  On/Off : Switch  Criteria=u2 > Threshold  Threshold=0.3
  Product{,1,3..4} (4 alike) : Product  RndMeth=Zero
  Product2 : Product  Inputs=*/  RndMeth=Zero
  Relational Operator : RelationalOperator  Operator=<  OutDataTypeStr=boolean
  Relational Operator1 : RelationalOperator  Operator=>  OutDataTypeStr=boolean
  "Reset " : InportShadow  Port=2
  Saturation Dynamic : simulink/Discontinuities/Saturation Dynamic  OutMin=[]  OutMax=[]  OutDataTypeStr=Inherit: Same as second input  OutDataType=fixdt(1, 16)  OutScaling=2^-10  DoSatur=off
  SaturationLimit : Constant  Value=upperSaturationLimit  OutDataTypeStr=single
  SaturationLimit1 : Constant  Value=lowerSaturationLimit  OutDataTypeStr=single
  Sum : Sum  Inputs=|+-
  Sum2 : Sum  Inputs=+++
  Trapezoidal Integrator : Subsystem  mask{T=Tsample}
      mask prompts: T "Sample Time"
  "Trim " : InportShadow  Port=4
  delayTime : Constant  Value=Ndelay*Tsample  OutDataTypeStr=single
  Output : Outport
  wires:
  On/Off/1 -> Memory1/1, Saturation Dynamic/2
  Constant1/1 -> On/Off/1
  "Reset "/1 -> On/Off/2
  Add2/1 -> On/Off/3
  [NotSaturated] -> AntiWindup/2
  Saturation Dynamic/1 -> Output/1
  Product2/1 -> Product3/1
  [Kd] -> Product3/2
  delayTime/1 -> Product2/2
  Sum/1 -> Product2/1
  NDelays/1 -> Sum/2
  [Kp] -> Product1/2
  Trapezoidal Integrator/1(Int(x)) -> Product/1
  [Ki] -> Product/2
  Error/1 -> Product1/1, Sum/1, NDelays/1, AntiWindup/1, Gain/1
  AntiWindup/1 -> Trapezoidal Integrator/1(x)
  Constant5/1 -> AntiWindup/3
  Demux/3 -> [Kd]
  Demux/2 -> [Ki]
  Demux/1 -> [Kp]
  PIDGains/1 -> Demux/1
  Memory1/1 -> [Out]
  Reset/1 -> Trapezoidal Integrator/2(Reset)
  Product1/1 -> Add1/1
  Product3/1 -> Add1/2
  Add1/1 -> [PDpart], Add2/1
  Product/1 -> Add2/2
  [PDpart] -> Sum2/3
  Product4/1 -> Sum2/1
  Gain/1 -> Product4/1
  [Ki] -> Product4/2
  Sum2/1 -> Relational Operator/1, Relational Operator1/1
  [Out] -> Sum2/2
  Add3/1 -> Relational Operator/2, [upLimit]
  Relational Operator/1 -> Logical Operator/2
  Relational Operator1/1 -> Logical Operator/1
  Logical Operator/1 -> [NotSaturated]
  Trim/1 -> Add3/2
  SaturationLimit/1 -> Add3/1
  Add4/1 -> Relational Operator1/2, [lowLimit]
  SaturationLimit1/1 -> Add4/1
  "Trim "/1 -> Add4/2
  [upLimit] -> Saturation Dynamic/1
  [lowLimit] -> Saturation Dynamic/3

== system AUAV_V3_TestSensors/Inner Loop// Navigation/Lateral Channel Encaps [updated 4.28.16]/Lateral Channel/psi_dot to Bank ==
  psi_dot_c : Inport
  U_m : Inport  Port=2
  Constant1 : Constant  Value=9.80665  OutDataTypeStr=single
  Divide : Product  Inputs=**/
  dsPIC_atan : Subsystem  AncestorBlock=SLUGS_Library/dsPIC_atan
  phi_c : Outport
  wires:
  Divide/1 -> dsPIC_atan/1(x)
  dsPIC_atan/1(atan(x)) -> phi_c/1
  Constant1/1 -> Divide/3
  U_m/1 -> Divide/2
  psi_dot_c/1 -> Divide/1

== system AUAV_V3_TestSensors/Inner Loop// Navigation/Lateral Channel Encaps [updated 4.28.16]/psi_dot_c Select logic1/Bank to Psi Dot ==
  phi_c : Inport
  U_m : Inport  Port=2
  Constant1 : Constant  Value=9.80665  OutDataTypeStr=single
  Divide : Product  Inputs=/*  OutDataTypeStr=single
  Divide1 : Product  OutDataTypeStr=single
  Protect NaNs : Subsystem
  Protect NaNs1 : Subsystem
  "[0 40]" : Saturate  UpperLimit=40  LowerLimit=0  SampleTime=.01
  bank Limit : Saturate  UpperLimit=bankCommandLimit  LowerLimit=-bankCommandLimit  SampleTime=.01
  dsPIC_tan : Subsystem  AncestorBlock=SLUGS_Library/dsPIC_tan
  psi_dot_c : Outport
  wires:
  "[0 40]"/1 -> Divide/1
  Divide/1 -> Divide1/2
  phi_c/1 -> Protect NaNs/1(In1)
  dsPIC_tan/1(tan(x)) -> Divide1/1
  Divide1/1 -> psi_dot_c/1
  Constant1/1 -> Divide/2
  U_m/1 -> Protect NaNs1/1(In1)
  bank Limit/1 -> dsPIC_tan/1(x)
  Protect NaNs/1(Out1) -> bank Limit/1
  Protect NaNs1/1(Out1) -> "[0 40]"/1

== system AUAV_V3_TestSensors/Inner Loop// Navigation/Longitudinal Channel Encaps [updated 4.28.16]/Longitudinal Channel/0.5 sec  tau for Turns ==
  In1 : Inport
  Constant : Constant  Value=T
  Constant1 : Constant  Value=f
  Embedded MATLAB Function : MATLAB Function  TreatAsAtomicUnit=on
  Out1 : Outport
  wires:
  Constant/1 -> Embedded MATLAB Function/2(T)
  Constant1/1 -> Embedded MATLAB Function/3(f)
  Embedded MATLAB Function/1(y) -> Out1/1
  In1/1 -> Embedded MATLAB Function/1(u)

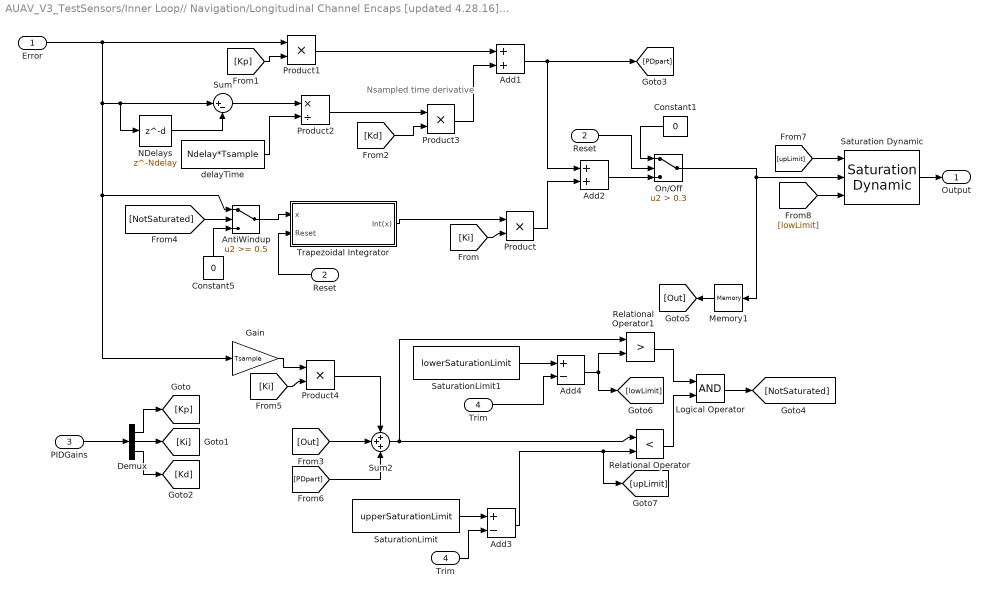
== system AUAV_V3_TestSensors/Inner Loop// Navigation/Longitudinal Channel Encaps [updated 4.28.16]/Longitudinal Channel/Airspeed Hold [PID] ==
  note: Nsampled time derivative
  Error : Inport
  Reset : Inport  Port=2
  PIDGains : Inport  Port=3
  Trim : Inport  Port=4
  Add1 : Sum
  Add2 : Sum  OutDataTypeStr=single
  Add3 : Sum  Inputs=+-  OutDataTypeStr=single
  Add4 : Sum  Inputs=+-  OutDataTypeStr=single
  AntiWindup : Switch  Threshold=0.5
  Constant1 : Constant  Value=0  OutDataTypeStr=single
  Constant5 : Constant  Value=0  OutDataTypeStr=single
  Demux : Demux  Outputs=3
  Gain : Gain  Gain=Tsample
  Logical Operator : Logic  AllPortsSameDT=off  OutDataTypeStr=boolean
  Memory1 : Memory  InheritSampleTime=on
  NDelays : Delay  DelayLength=Ndelay  InputProcessing=Inherited  SampleTime=Tsample
  On/Off : Switch  Criteria=u2 > Threshold  Threshold=0.3
  Product{,1,3..4} (4 alike) : Product  RndMeth=Zero
  Product2 : Product  Inputs=*/  RndMeth=Zero
  Relational Operator : RelationalOperator  Operator=<  OutDataTypeStr=boolean
  Relational Operator1 : RelationalOperator  Operator=>  OutDataTypeStr=boolean
  "Reset " : InportShadow  Port=2
  Saturation Dynamic : simulink/Discontinuities/Saturation Dynamic  OutMin=[]  OutMax=[]  OutDataTypeStr=Inherit: Same as second input  OutDataType=fixdt(1, 16)  OutScaling=2^-10  DoSatur=off
  SaturationLimit : Constant  Value=upperSaturationLimit  OutDataTypeStr=single
  SaturationLimit1 : Constant  Value=lowerSaturationLimit  OutDataTypeStr=single
  Sum : Sum  Inputs=|+-
  Sum2 : Sum  Inputs=+++
  Trapezoidal Integrator : Subsystem  mask{T=Tsample}
      mask prompts: T "Sample Time"
  "Trim " : InportShadow  Port=4
  delayTime : Constant  Value=Ndelay*Tsample  OutDataTypeStr=single
  Output : Outport
  wires:
  On/Off/1 -> Memory1/1, Saturation Dynamic/2
  Constant1/1 -> On/Off/1
  "Reset "/1 -> On/Off/2
  Add2/1 -> On/Off/3
  [NotSaturated] -> AntiWindup/2
  Saturation Dynamic/1 -> Output/1
  Product2/1 -> Product3/1
  [Kd] -> Product3/2
  delayTime/1 -> Product2/2
  Sum/1 -> Product2/1
  NDelays/1 -> Sum/2
  [Kp] -> Product1/2
  Trapezoidal Integrator/1(Int(x)) -> Product/1
  [Ki] -> Product/2
  Error/1 -> Product1/1, Sum/1, NDelays/1, AntiWindup/1, Gain/1
  AntiWindup/1 -> Trapezoidal Integrator/1(x)
  Constant5/1 -> AntiWindup/3
  Demux/3 -> [Kd]
  Demux/2 -> [Ki]
  Demux/1 -> [Kp]
  PIDGains/1 -> Demux/1
  Memory1/1 -> [Out]
  Reset/1 -> Trapezoidal Integrator/2(Reset)
  Product1/1 -> Add1/1
  Product3/1 -> Add1/2
  Add1/1 -> [PDpart], Add2/1
  Product/1 -> Add2/2
  [PDpart] -> Sum2/3
  Product4/1 -> Sum2/1
  Gain/1 -> Product4/1
  [Ki] -> Product4/2
  Sum2/1 -> Relational Operator/1, Relational Operator1/1
  [Out] -> Sum2/2
  Add3/1 -> Relational Operator/2, [upLimit]
  Relational Operator/1 -> Logical Operator/2
  Relational Operator1/1 -> Logical Operator/1
  Logical Operator/1 -> [NotSaturated]
  Trim/1 -> Add3/2
  SaturationLimit/1 -> Add3/1
  Add4/1 -> Relational Operator1/2, [lowLimit]
  SaturationLimit1/1 -> Add4/1
  "Trim "/1 -> Add4/2
  [upLimit] -> Saturation Dynamic/1
  [lowLimit] -> Saturation Dynamic/3

== system AUAV_V3_TestSensors/Inner Loop// Navigation/Longitudinal Channel Encaps [updated 4.28.16]/Longitudinal Channel/Height Error to Pitch Command [PI] ==
  Error : Inport
  Reset : Inport  Port=2
  PIDGains : Inport  Port=3
  Trim : Inport  Port=4
  Add2 : Sum  OutDataTypeStr=single
  Add3 : Sum  Inputs=+-  OutDataTypeStr=single
  Add4 : Sum  Inputs=+-  OutDataTypeStr=single
  AntiWindup : Switch  Threshold=0.5
  Constant1 : Constant  Value=0  OutDataTypeStr=single
  Constant5 : Constant  Value=0  OutDataTypeStr=single
  Demux : Demux  Outputs=2
  Gain : Gain  Gain=Tsample
  Logical Operator : Logic  AllPortsSameDT=off  OutDataTypeStr=boolean
  Memory1 : Memory  InheritSampleTime=on
  On/Off : Switch  Criteria=u2 > Threshold  Threshold=0.3
  Product : Product  RndMeth=Zero
  Product1 : Product  RndMeth=Zero
  Product4 : Product  RndMeth=Zero
  Relational Operator : RelationalOperator  Operator=<  OutDataTypeStr=boolean
  Relational Operator1 : RelationalOperator  Operator=>  OutDataTypeStr=boolean
  "Reset " : InportShadow  Port=2
  Saturation Dynamic : simulink/Discontinuities/Saturation Dynamic  OutMin=[]  OutMax=[]  OutDataTypeStr=Inherit: Same as second input  OutDataType=fixdt(1, 16)  OutScaling=2^-10  DoSatur=off
  SaturationLimit : Constant  Value=upperSaturationLimit  OutDataTypeStr=single
  SaturationLimit1 : Constant  Value=lowerSaturationLimit  OutDataTypeStr=single
  Sum2 : Sum  Inputs=+++
  Trapezoidal Integrator : Subsystem  mask{T=Tsample}
      mask prompts: T "Sample Time"
  "Trim " : InportShadow  Port=4
  Output : Outport
  wires:
  On/Off/1 -> Memory1/1, Saturation Dynamic/2
  Constant1/1 -> On/Off/1
  "Reset "/1 -> On/Off/2
  Add2/1 -> On/Off/3
  [lowLimit] -> Saturation Dynamic/3
  [upLimit] -> Saturation Dynamic/1
  "Trim "/1 -> Add4/2
  SaturationLimit1/1 -> Add4/1
  Add4/1 -> [lowLimit], Relational Operator1/2
  SaturationLimit/1 -> Add3/1
  Trim/1 -> Add3/2
  Logical Operator/1 -> [NotSaturated]
  Relational Operator1/1 -> Logical Operator/1
  Relational Operator/1 -> Logical Operator/2
  Add3/1 -> [upLimit], Relational Operator/2
  [Out] -> Sum2/2
  Sum2/1 -> Relational Operator1/1, Relational Operator/1
  [Ki] -> Product4/2
  Gain/1 -> Product4/1
  Product4/1 -> Sum2/1
  [PDpart] -> Sum2/3
  Product/1 -> Add2/2
  Product1/1 -> Add2/1, [PDpart]
  Reset/1 -> Trapezoidal Integrator/2(Reset)
  Memory1/1 -> [Out]
  PIDGains/1 -> Demux/1
  Demux/1 -> [Kp]
  Demux/2 -> [Ki]
  Constant5/1 -> AntiWindup/3
  AntiWindup/1 -> Trapezoidal Integrator/1(x)
  Error/1 -> Product1/1, Gain/1, AntiWindup/1
  [Ki] -> Product/2
  Trapezoidal Integrator/1(Int(x)) -> Product/1
  [Kp] -> Product1/2
  Saturation Dynamic/1 -> Output/1
  [NotSaturated] -> AntiWindup/2

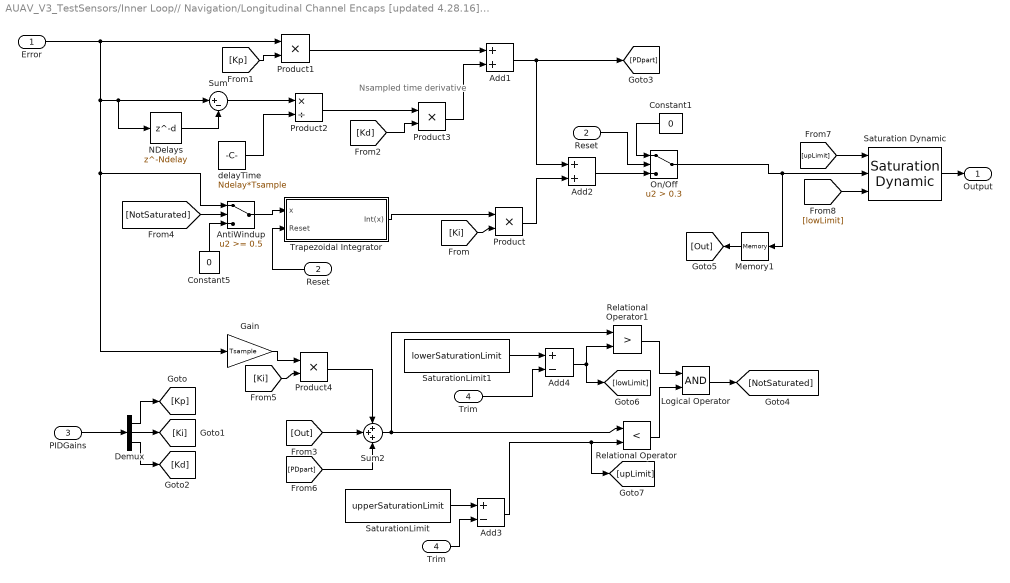
== system AUAV_V3_TestSensors/Inner Loop// Navigation/Longitudinal Channel Encaps [updated 4.28.16]/Longitudinal Channel/Pitch To Elevator [PID] ==
  note: Nsampled time derivative
  Error : Inport
  Reset : Inport  Port=2
  PIDGains : Inport  Port=3
  Trim : Inport  Port=4
  Add1 : Sum
  Add2 : Sum  OutDataTypeStr=single
  Add3 : Sum  Inputs=+-  OutDataTypeStr=single
  Add4 : Sum  Inputs=+-  OutDataTypeStr=single
  AntiWindup : Switch  Threshold=0.5
  Constant1 : Constant  Value=0  OutDataTypeStr=single
  Constant5 : Constant  Value=0  OutDataTypeStr=single
  Demux : Demux  Outputs=3
  Gain : Gain  Gain=Tsample
  Logical Operator : Logic  AllPortsSameDT=off  OutDataTypeStr=boolean
  Memory1 : Memory  InheritSampleTime=on
  NDelays : Delay  DelayLength=Ndelay  InputProcessing=Inherited  SampleTime=Tsample
  On/Off : Switch  Criteria=u2 > Threshold  Threshold=0.3
  Product{,1,3..4} (4 alike) : Product  RndMeth=Zero
  Product2 : Product  Inputs=*/  RndMeth=Zero
  Relational Operator : RelationalOperator  Operator=<  OutDataTypeStr=boolean
  Relational Operator1 : RelationalOperator  Operator=>  OutDataTypeStr=boolean
  "Reset " : InportShadow  Port=2
  Saturation Dynamic : simulink/Discontinuities/Saturation Dynamic  OutMin=[]  OutMax=[]  OutDataTypeStr=Inherit: Same as second input  OutDataType=fixdt(1, 16)  OutScaling=2^-10  DoSatur=off
  SaturationLimit : Constant  Value=upperSaturationLimit  OutDataTypeStr=single
  SaturationLimit1 : Constant  Value=lowerSaturationLimit  OutDataTypeStr=single
  Sum : Sum  Inputs=|+-
  Sum2 : Sum  Inputs=+++
  Trapezoidal Integrator : Subsystem  mask{T=Tsample}
      mask prompts: T "Sample Time"
  "Trim " : InportShadow  Port=4
  delayTime : Constant  Value=Ndelay*Tsample  OutDataTypeStr=single
  Output : Outport
  wires:
  On/Off/1 -> Memory1/1, Saturation Dynamic/2
  Constant1/1 -> On/Off/1
  "Reset "/1 -> On/Off/2
  Add2/1 -> On/Off/3
  [NotSaturated] -> AntiWindup/2
  Saturation Dynamic/1 -> Output/1
  Product2/1 -> Product3/1
  [Kd] -> Product3/2
  delayTime/1 -> Product2/2
  Sum/1 -> Product2/1
  NDelays/1 -> Sum/2
  [Kp] -> Product1/2
  Trapezoidal Integrator/1(Int(x)) -> Product/1
  [Ki] -> Product/2
  Error/1 -> Product1/1, Sum/1, NDelays/1, AntiWindup/1, Gain/1
  AntiWindup/1 -> Trapezoidal Integrator/1(x)
  Constant5/1 -> AntiWindup/3
  Demux/3 -> [Kd]
  Demux/2 -> [Ki]
  Demux/1 -> [Kp]
  PIDGains/1 -> Demux/1
  Memory1/1 -> [Out]
  Reset/1 -> Trapezoidal Integrator/2(Reset)
  Product1/1 -> Add1/1
  Product3/1 -> Add1/2
  Add1/1 -> [PDpart], Add2/1
  Product/1 -> Add2/2
  [PDpart] -> Sum2/3
  Product4/1 -> Sum2/1
  Gain/1 -> Product4/1
  [Ki] -> Product4/2
  Sum2/1 -> Relational Operator/1, Relational Operator1/1
  [Out] -> Sum2/2
  Add3/1 -> Relational Operator/2, [upLimit]
  Relational Operator/1 -> Logical Operator/2
  Relational Operator1/1 -> Logical Operator/1
  Logical Operator/1 -> [NotSaturated]
  Trim/1 -> Add3/2
  SaturationLimit/1 -> Add3/1
  Add4/1 -> Relational Operator1/2, [lowLimit]
  SaturationLimit1/1 -> Add4/1
  "Trim "/1 -> Add4/2
  [upLimit] -> Saturation Dynamic/1
  [lowLimit] -> Saturation Dynamic/3

== system AUAV_V3_TestSensors/Inner Loop// Navigation/Longitudinal Channel Encaps [updated 4.28.16]/Longitudinal Channel/Pitot Control End ==
  dyn P [Pa] : Inport
  H_m [m] : Inport  Port=2
  " 0.3 sec tau for high speeds" : Subsystem  mask(Tustin1stOrderLowpassAutoInitialCondition){f=1, T=T}
      mask prompts: f "Lowpass Frequency"; T "Sample Time"
      mask help: Takes a 3db rolloff frequency (in Hz, NOT radians/s) and a sample time. Performs a symbolic Tustin conversion and implements in a discrete filter. The initial output of the filter is set by the first sample.
      mask Help: Enter the desired 3db rolloff frequency in Hz and the sample time. Initial conditions are sampled automatically.
      mask Display: fprintf('%.2f Hz lowpass',f)
  Air Density from Height : Subsystem
  Compute Airspeed : Subsystem
  Protect NaN : Subsystem
  Schedule LPF : Switch  Criteria=u2 > Threshold  Threshold=0.3  OutDataTypeStr=single
  lowpass limit : simulink/Logic and Bit Operations/Compare To Constant  relop=<=  const=5  OutDataTypeStr=uint8  ZeroCross=off
  AirSpeed[m/s] : Outport
  wires:
  H_m [m]/1 -> Air Density from Height/1(h(m))
  Schedule LPF/1 -> AirSpeed[m/s]/1
  dyn P [Pa]/1 -> Compute Airspeed/1(Dyn P)
  Air Density from Height/1(rho (Kg/m^3)) -> Compute Airspeed/2(rho)
  Compute Airspeed/1(Airspeed m(s)) -> Protect NaN/1(In1)
  lowpass limit/1 -> Schedule LPF/2
  " 0.3 sec tau for high speeds"/1(Out1) -> Schedule LPF/3
  Protect NaN/1(Out1) -> " 0.3 sec tau for high speeds"/1(In1), lowpass limit/1, Schedule LPF/1

== system AUAV_V3_TestSensors/Inner Loop// Navigation/Longitudinal Channel Encaps [updated 4.28.16]/Longitudinal Channel/Protect NaNs ==
  In1 : Inport
  Integer Delay3 : Delay  DelayLength=1  InputProcessing=Inherited  SampleTime=T
  Relational Operator2 : RelationalOperator  Operator===  OutDataTypeStr=uint(8)
  Switch3 : Switch  Criteria=u2 > Threshold  Threshold=0.3  SampleTime=.01
  Out1 : Outport
  wires:
  Integer Delay3/1 -> Switch3/3
  Switch3/1 -> Out1/1, Integer Delay3/1
  In1/1 -> Relational Operator2/2, Relational Operator2/1, Switch3/1
  Relational Operator2/1 -> Switch3/2

== system AUAV_V3_TestSensors/Inner Loop// Navigation/Longitudinal Channel Encaps [updated 4.28.16]/Longitudinal Channel/Protect NaNs1 ==
  In1 : Inport
  Integer Delay3 : Delay  DelayLength=1  InputProcessing=Inherited  SampleTime=T
  Relational Operator2 : RelationalOperator  Operator===  OutDataTypeStr=uint(8)
  Switch3 : Switch  Criteria=u2 > Threshold  Threshold=0.3  SampleTime=.01
  Out1 : Outport
  wires:
  Integer Delay3/1 -> Switch3/3
  Switch3/1 -> Out1/1, Integer Delay3/1
  In1/1 -> Relational Operator2/2, Relational Operator2/1, Switch3/1
  Relational Operator2/1 -> Switch3/2

== system AUAV_V3_TestSensors/Inner Loop// Navigation/Longitudinal Channel Encaps [updated 4.28.16]/Longitudinal Channel/Protect NaNs2 ==
  In1 : Inport
  Integer Delay3 : Delay  DelayLength=1  InputProcessing=Inherited  SampleTime=T
  Relational Operator2 : RelationalOperator  Operator===  OutDataTypeStr=uint(8)
  Switch3 : Switch  Criteria=u2 > Threshold  Threshold=0.3  SampleTime=.01
  Out1 : Outport
  wires:
  Relational Operator2/1 -> Switch3/2
  In1/1 -> Switch3/1, Relational Operator2/1, Relational Operator2/2
  Switch3/1 -> Integer Delay3/1, Out1/1
  Integer Delay3/1 -> Switch3/3

== system AUAV_V3_TestSensors/Inner Loop// Navigation/Longitudinal Channel Encaps [updated 4.28.16]/Longitudinal Channel/Protect NaNs4 ==
  In1 : Inport
  Integer Delay3 : Delay  DelayLength=1  InputProcessing=Inherited  SampleTime=T
  Relational Operator2 : RelationalOperator  Operator===  OutDataTypeStr=uint(8)
  Switch3 : Switch  Criteria=u2 > Threshold  Threshold=0.3  SampleTime=.01
  Out1 : Outport
  wires:
  Relational Operator2/1 -> Switch3/2
  In1/1 -> Switch3/1, Relational Operator2/1, Relational Operator2/2
  Switch3/1 -> Integer Delay3/1, Out1/1
  Integer Delay3/1 -> Switch3/3

== system AUAV_V3_TestSensors/Inner Loop// Navigation/Longitudinal Channel Encaps [updated 4.28.16]/Longitudinal Channel/dsPIC_cos ==
  u : Inport
  Environment Controller1 : simulink/Signal Routing/Environment Controller
  Trigonometric Function : Trigonometry  Operator=cos
  myCos() apUtils.c [updated 5.1.16] : MCHP_Blockset/User Functions/C Function Call  ParseFilesChkbx=off  ListFunctions1=Custom Function  Function1=float myCos(float x)  AddHeaderDeclaration=off  Function1Type=when block is updated (default)  Fct1BlockIn=x  FctReturnBlockOut=on  DataCollected=0  ORDERING=None  SampleTime=-1  MCHP_MASTERLINK=|  PinDigitalInput=[]  PinDigitalOutput=[]  PinAnalogInput=[]
      | AUAV_V3_TestSensors/Microchip Master
      | AUAV V3 Board
      | Busy Flag on D2 (RA6)
  cos(u) : Outport
  wires:
  u/1 -> Trigonometric Function/1, myCos() apUtils.c [updated 5.1.16]/1
  Environment Controller1/1 -> cos(u)/1
  myCos() apUtils.c [updated 5.1.16]/1 -> Environment Controller1/2
  Trigonometric Function/1 -> Environment Controller1/1
